simulink model "SignalSurPorteuse"  (Simulink 10.1)
settings: Solver=VariableStepAuto  StartTime=0.0  StopTime=2000/9e6  RelTol=1e-3
libraries: commrandsrc3 x1, commdigbbndam3 x1, dspsrcs4 x1
settings Model: Creator=iba  LastModifiedBy=iba
settings DataIOCC: SaveFormat=Dataset  ReturnWorkspaceOutputs=on
settings OptimizationCC: LifeSpan=auto
settings DebuggingCC: UnderspecifiedInitializationDetection=Simplified  MergeDetectMultiDrivingBlocksExec=error  SFUnexpectedBacktrackingDiag=error  SFNoUnconditionalDefaultTransitionDiag=error  SFExecutionAtInitializationDiag=warning  ArithmeticOperatorsInVariantConditions=error
settings HardwareCC: ProdBitPerPointer=64  ProdBitPerSizeT=64  ProdBitPerPtrDiffT=64  ProdLargestAtomicFloat=Float  ProdIntDivRoundTo=Zero  ProdEndianess=LittleEndian  ProdWordSize=64  ProdHWDeviceType=Intel->x86-64 (Windows64)
settings ModelReferenceCC: PropagateSignalLabelsOutOfModel=on
settings SFSimCC: SimUseLocalCustomCode=on  CustomCodeUndefinedFunction=FilterOut
settings RTWCC: RTWUseLocalCustomCode=on
settings CodeAppCC: StateflowObjectComments=off
settings GRTTargetCC: TargetLangStandard=C99 (ISO)  CombineOutputUpdateFcns=on  GRTInterface=off
settings ConfigComp: CovMetricSettings=dwe  CovHtmlReporting=off  CovSaveCumulativeToWorkspaceVar=off  CovSaveSingleToWorkspaceVar=off  CovExternalEMLEnable=on

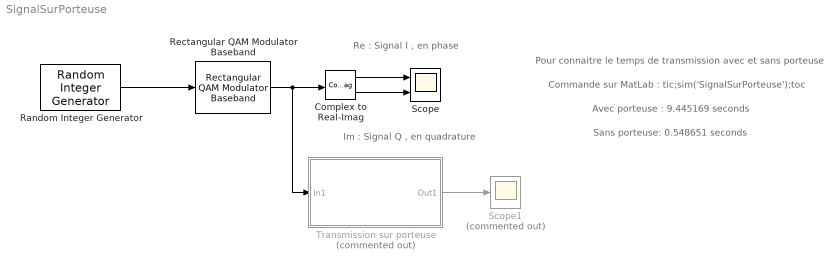
== system SignalSurPorteuse ==
  note: Sans porteuse: 0.548651 seconds
  note: Avec porteuse : 9.445169 seconds
  note: Pour connaitre le temps de transmission avec et sans porteuse
  note: Commande sur MatLab : tic;sim('SignalSurPorteuse');toc
  note: Re : Signal I , en phase
  note: Im : Signal Q , en quadrature
  Complex to Real-Imag : ComplexToRealImag
  Random Integer Generator : commrandsrc3/Random Integer Generator  SetSize=64  SeedSource=Parameter  Seed=37  SampleTime=1/9e6  SamplesPerFrame=1  OutputDataType=double  SimulateUsing=Interpreted execution
  Rectangular QAM Modulator Baseband : commdigbbndam3/Rectangular QAM Modulator Baseband  M=64  InType=Integer  Enc=Gray  Mapping=[0:15]  PowType=Min. distance between symbols  MinDist=2  AvgPow=1  PeakPow=1  Ph=0  outDtype=double  outWordLen=16  outUDDataType=sfix(16)  outFracLenMode=Best precision  outFracLen=15  outDataTypeStr=double  outLastDataTypeStr=double
  Scope : Scope  NumInputPorts=2
  Scope1 : Scope  Commented=on
  Transmission sur porteuse : Subsystem  Commented=on  mask(Utilitaire pour les communications){Fo=5e9, Ts=1/10.5e9}
      mask prompts: Fo "Fréquence de la porteuse (Hz)"; Ts "Pas d'échantillonnage (s)"
      mask help: Transforme le signal complexe en bande de base en un signal réel sur porteuse.
      mask Display: disp('Transmission sur porteuse')
  wires:
  Random Integer Generator/1 -> Rectangular QAM Modulator Baseband/1
  Rectangular QAM Modulator Baseband/1 -> Transmission sur porteuse/1(In1), Complex to Real-Imag/1
  Complex to Real-Imag/1 -> Scope/1
  Complex to Real-Imag/2 -> Scope/2
  Transmission sur porteuse/1(Out1) -> Scope1/1

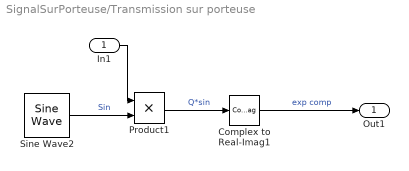
== system SignalSurPorteuse/Transmission sur porteuse ==
  In1 : Inport
  Complex to Real-Imag1 : ComplexToRealImag  Output=Real
  Product1 : Product
  Sine Wave2 : dspsrcs4/Sine Wave  Amplitude=1  Frequency=Fo  Phase=0  SampleMode=Discrete  OutComplex=Complex  CompMethod=Trigonometric fcn  TableSize=Speed  SampleTime=Ts  SamplesPerFrame=1  ResetState=Restart at time zero  OutputFrames=off  dataType=double  wordLen=16  udDataType=sfix(16)  fracBitsMode=Best precision  numFracBits=15  OutDataTypeStr=double  LastOutDataTypeStr=double
  Out1 : Outport
  wires:
  Sine Wave2/1 -> Product1/2  "Sin"
  Complex to Real-Imag1/1 -> Out1/1  "exp comp"
  Product1/1 -> Complex to Real-Imag1/1  "Q*sin"
  In1/1 -> Product1/1
